simulink model "Stage"  (R2019b)
settings: Solver=ode8  StartTime=0.0  StopTime=0.101  FixedStep=1/6e4  RelTol=1e-3
libraries: simulink x1
settings Model: Creator=cwh  LastModifiedBy=cwh

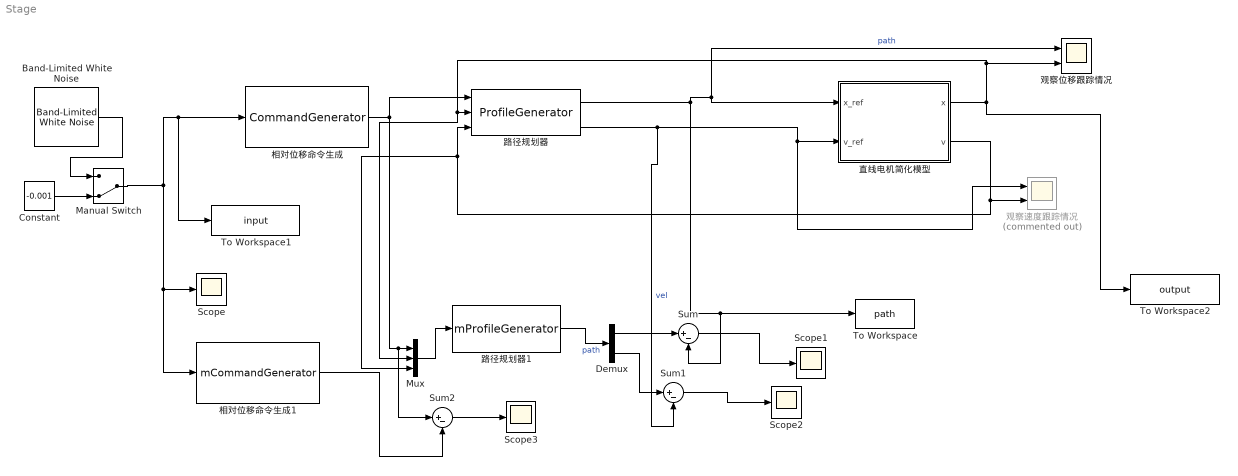
== system Stage ==
  Band-Limited White Noise : simulink/Sources/Band-Limited White Noise  Cov=[0.00000000001]  Ts=1/300  seed=[724534]
  Constant : Constant  Value=-0.001
  Demux : Demux  Outputs=2
  Manual Switch : ManualSwitch  CurrentSetting=0
  Mux : Mux  Inputs=3
  Scope{,1..3} (4 alike) : Scope
  Sum : Sum  Inputs=|+-
  Sum1 : Sum  Inputs=|+-
  Sum2 : Sum  Inputs=|+-
  To Workspace : ToWorkspace  VariableName=path  SampleTime=-1
      settings: Save2DSignal=2-D array (concatenate along first dimension)
  To Workspace1 : ToWorkspace  VariableName=input  SampleTime=1/300
      settings: Save2DSignal=2-D array (concatenate along first dimension)
  To Workspace2 : ToWorkspace  VariableName=output  SampleTime=1/300
      settings: Save2DSignal=2-D array (concatenate along first dimension)
  直线电机简化模型 : Subsystem  mask{ts=5e-5, L=1.94e-3, R=2.46, Ki=4.6, Kf=0, Kbemf=2.81, M=1, Kpx=15, Kix=0.001, Kdx=0.02, Kpv=0.05, Kiv=0.5, Kdv=0, Kpi=5, Kii=0.0015, Kdi=0}
      mask prompts: ts "Control period"; L "Coil inductance"; R "Coil resistance"; Ki "Force coefficient"; Kf "Friction coefficient"; Kbemf "Back EMF Coefficient"; M "Moving mass"; Kpx "Kp in position loop"; Kix "Ki in position loop"; Kdx "Kd in position loop"; Kpv "Kp in velocity loop"; Kiv "Ki in velocity lpop"; Kdv "Kd in velocity loop"; Kpi "Kp in current loop"; Kii "Ki in current loop"; Kdi "Kd in current loop"
  相对位移命令生成 : S-Function  FunctionName=CommandGenerator  Parameters=ts0,cp0  SFunctionDeploymentMode=off  EnableBusSupport=off  mask{ts0=5e-5, cp0=1/300}
      mask prompts: ts0 "Serving period"; cp0 "Command period"
  相对位移命令生成1 : S-Function  FunctionName=mCommandGenerator  Parameters=ts0,cp0  SFunctionDeploymentMode=off  EnableBusSupport=off  mask{ts0=5e-5, cp0=1/300}
      mask prompts: ts0 "Serving period"; cp0 "Command period"
  观察位移跟踪情况 : Scope  NumInputPorts=2
  观察速度跟踪情况 : Scope  Commented=on  NumInputPorts=2
  路径规划器 : S-Function  FunctionName=ProfileGenerator  Parameters=ts0,vmax0,amax0  SFunctionDeploymentMode=off  EnableBusSupport=off  mask{ts0=5e-5, vmax0=0.5, amax0=3}
      mask prompts: ts0 "Control period"; vmax0 "Max velocity"; amax0 "Max acceleration"
  路径规划器1 : S-Function  FunctionName=mProfileGenerator  Parameters=ts0,vmax0,amax0  SFunctionDeploymentMode=off  EnableBusSupport=off  mask{ts0=5e-5, vmax0=0.5, amax0=3}
      mask prompts: ts0 "Control period"; vmax0 "Max velocity"; amax0 "Max acceleration"
  wires:
  相对位移命令生成/1 -> Sum2/1, Mux/1, 路径规划器/1
  直线电机简化模型/1(x) -> Mux/2, 路径规划器/2, 观察位移跟踪情况/2, To Workspace2/1
  直线电机简化模型/2(v) -> Mux/3, 路径规划器/3, 观察速度跟踪情况/2
  路径规划器/1 -> 观察位移跟踪情况/1, 直线电机简化模型/1(x_ref), Sum/2, To Workspace/1  "path"
  路径规划器/2 -> Sum1/2, 观察速度跟踪情况/1, 直线电机简化模型/2(v_ref)  "vel"
  Manual Switch/1 -> 相对位移命令生成1/1, Scope/1, 相对位移命令生成/1, To Workspace1/1
  Constant/1 -> Manual Switch/2
  Band-Limited White Noise/1 -> Manual Switch/1
  路径规划器1/1 -> Demux/1  "path"
  Demux/1 -> Sum/1
  Demux/2 -> Sum1/1
  Sum/1 -> Scope1/1
  Mux/1 -> 路径规划器1/1
  Sum1/1 -> Scope2/1
  相对位移命令生成1/1 -> Sum2/2
  Sum2/1 -> Scope3/1

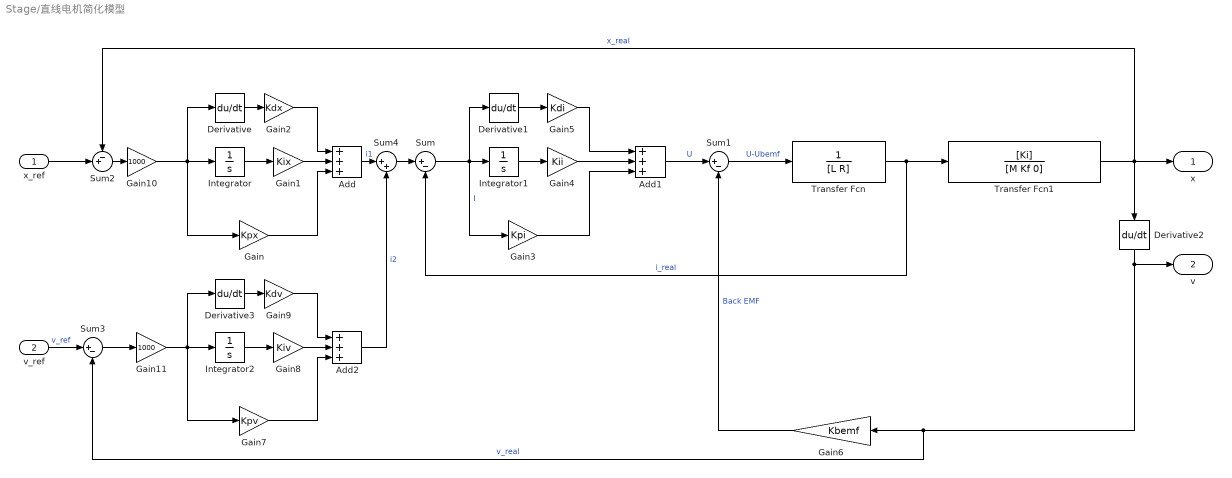
== system Stage/直线电机简化模型 ==
  x_ref : Inport
  v_ref : Inport  Port=2
  Add : Sum  Inputs=+++
  Add1 : Sum  Inputs=+++
  Add2 : Sum  Inputs=+++
  Derivative{,1..3} (4 alike) : Derivative
  Gain : Gain  Gain=Kpx
  Gain1 : Gain  Gain=Kix
  Gain10 : Gain  Gain=1000
  Gain11 : Gain  Gain=1000
  Gain2 : Gain  Gain=Kdx
  Gain3 : Gain  Gain=Kpi
  Gain4 : Gain  Gain=Kii
  Gain5 : Gain  Gain=Kdi
  Gain6 : Gain  Gain=Kbemf
  Gain7 : Gain  Gain=Kpv
  Gain8 : Gain  Gain=Kiv
  Gain9 : Gain  Gain=Kdv
  Integrator : Integrator
  Integrator1 : Integrator
  Integrator2 : Integrator
  Sum : Sum  Inputs=|+-
  Sum1 : Sum  Inputs=|+-
  Sum2 : Sum  Inputs=-+|
  Sum3 : Sum  Inputs=|+-
  Sum4 : Sum  Inputs=|++
  Transfer Fcn : TransferFcn  Denominator=[L R]
  Transfer Fcn1 : TransferFcn  Numerator=[Ki]  Denominator=[M Kf 0]
  x : Outport
  v : Outport  Port=2
  wires:
  Gain10/1 -> Derivative/1, Gain/1, Integrator/1
  Derivative/1 -> Gain2/1
  Integrator/1 -> Gain1/1
  Gain2/1 -> Add/1
  Gain1/1 -> Add/2
  Gain/1 -> Add/3
  Sum/1 -> Derivative1/1, Gain3/1, Integrator1/1  "I"
  Gain3/1 -> Add1/3
  Gain4/1 -> Add1/2
  Integrator1/1 -> Gain4/1
  Gain5/1 -> Add1/1
  Derivative1/1 -> Gain5/1
  Add1/1 -> Sum1/1  "U"
  Transfer Fcn/1 -> Transfer Fcn1/1, Sum/2  "i_real"
  Sum1/1 -> Transfer Fcn/1  "U-Ubemf"
  Transfer Fcn1/1 -> x/1, Sum2/1, Derivative2/1  "x_reaI"
  Derivative2/1 -> v/1, Sum3/2, Gain6/1  "v_real"
  Gain6/1 -> Sum1/2  "Back EMF"
  Gain7/1 -> Add2/3
  Gain11/1 -> Derivative3/1, Gain7/1, Integrator2/1
  Gain8/1 -> Add2/2
  Integrator2/1 -> Gain8/1
  Add2/1 -> Sum4/2  "i2"
  Gain9/1 -> Add2/1
  Derivative3/1 -> Gain9/1
  v_ref/1 -> Sum3/1  "v_ref"
  Add/1 -> Sum4/1  "i1"
  Sum4/1 -> Sum/1
  x_ref/1 -> Sum2/2
  Sum3/1 -> Gain11/1
  Sum2/1 -> Gain10/1
